simulink model "fu_simu_png_radome_directerror"  (R2020a)
settings: Solver=FixedStepAuto  StartTime=0.0  StopTime=20  FixedStep=0.001  RelTol=1e-3
values from neighbouring files (symbols this model uses):
  gamma_M_0 = deg2rad(0)    [initial.m]
  lambda_0 = deg2rad(5.7106)    [initial.m]
  N = 4    [initial.m]
  R_0 = 10050    [initial.m]
  T_alpha = 1    [initial.m]
  tau = 0.1    [initial.m]
  V_M = 500    [initial.m]
settings Model: Creator=anwaei  LastModifiedBy=anwaei

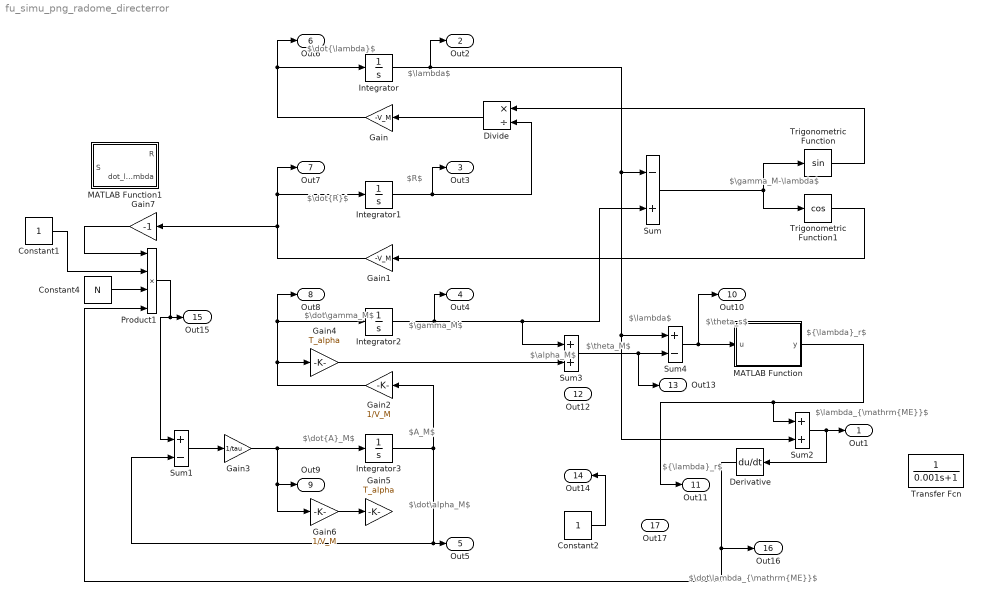
== system fu_simu_png_radome_directerror ==
  note: $\lambda$
  note: $R$
  note: $\gamma_M$
  note: $A_M$
  note: $\gamma_M-\lambda$
  note: $\dot{\lambda}$
  note: $\dot{R}$
  note: $\dot\gamma_M$
  note: $\dot{A}_M$
  note: $\alpha_M$
  note: $\theta_M$
  note: $\theta_s$
  note: $\dot\alpha_M$
  note: $\lambda$
  note: ${\lambda}_r$
  note: $\lambda_{\mathrm{ME}}$
  note: $\dot\lambda_{\mathrm{ME}}$
  note: ${\lambda}_r$
  Constant1 : Constant
  Constant2 : Constant
  Constant4 : Constant  Value=N
  Derivative : Derivative
  Divide : Product  Inputs=*/
  Gain : Gain  Gain=-V_M
  Gain1 : Gain  Gain=-V_M
  Gain2 : Gain  Gain=1/V_M
  Gain3 : Gain  Gain=1/tau
  Gain4 : Gain  Gain=T_alpha
  Gain5 : Gain  Gain=T_alpha
  Gain6 : Gain  Gain=1/V_M
  Gain7 : Gain  Gain=-1
  Integrator : Integrator  InitialCondition=lambda_0
  Integrator1 : Integrator  InitialCondition=R_0
  Integrator2 : Integrator  InitialCondition=gamma_M_0
  Integrator3 : Integrator
  MATLAB Function : MATLAB Function  TreatAsAtomicUnit=on
  MATLAB Function1 : MATLAB Function  TreatAsAtomicUnit=on
  Product1 : Product  Inputs=4
  Sum : Sum  Inputs=-+
  Sum1 : Sum  Inputs=+-
  Sum2 : Sum
  Sum3 : Sum
  Sum4 : Sum  Inputs=+-
  Transfer Fcn : TransferFcn  Denominator=[0.001 1]
  Trigonometric Function : Trigonometry
  Trigonometric Function1 : Trigonometry  Operator=cos
  Out1 : Outport
  Out2 : Outport  Port=2
  Out3 : Outport  Port=3
  Out4 : Outport  Port=4
  Out5 : Outport  Port=5
  Out6 : Outport  Port=6
  Out7 : Outport  Port=7
  Out8 : Outport  Port=8
  Out9 : Outport  Port=9
  Out10 : Outport  Port=10
  Out11 : Outport  Port=11
  Out12 : Outport  Port=12
  Out13 : Outport  Port=13
  Out14 : Outport  Port=14
  Out15 : Outport  Port=15
  Out16 : Outport  Port=16
  Out17 : Outport  Port=17
  wires:
  Integrator/1 -> Out2/1, Sum2/2, Sum4/1, Sum/1
  Integrator1/1 -> Out3/1, Divide/2
  Integrator2/1 -> Out4/1, Sum3/1, Sum/2
  Integrator3/1 -> Gain2/1, Sum1/2, Out5/1
  Sum/1 -> Trigonometric Function/1, Trigonometric Function1/1
  Trigonometric Function/1 -> Divide/1
  Divide/1 -> Gain/1
  Gain/1 -> Out6/1, Integrator/1
  Trigonometric Function1/1 -> Gain1/1
  Gain1/1 -> Gain7/1, Out7/1, Integrator1/1
  Gain2/1 -> Gain4/1, Out8/1, Integrator2/1
  Gain3/1 -> Out9/1, Gain6/1, Integrator3/1
  Sum3/1 -> Out13/1, Sum4/2
  Sum4/1 -> Out10/1, MATLAB Function/1(u)
  Gain6/1 -> Gain5/1
  MATLAB Function/1(y) -> Sum2/1, Out11/1
  Gain7/1 -> Product1/1
  Constant4/1 -> Product1/3
  Product1/1 -> Sum1/1, Out15/1
  Sum1/1 -> Gain3/1
  Sum2/1 -> Derivative/1, Out1/1
  Constant1/1 -> Product1/2
  Gain4/1 -> Sum3/2
  Derivative/1 -> Out16/1, Product1/4
  Constant2/1 -> Out14/1

== matlab function fu_simu_png_radome_directerror/MATLAB Function ==
  data: u input; y output
function y = fcn(u)

%%
r=deg2rad(-0.5);
zeta=4;
p=1;
y=r*exp(-zeta*abs(u))*sin(2*pi/p*u);

% if u<0
%     a=exp(zeta*u);
%     b=zeta*sin(2*pi*u/p);
%     c=2*pi/p*cos(2*pi*u/p);
% else
%     a=exp(-zeta*u);
%     b=-zeta*sin(2*pi*u/p);
%     c=2*pi/p*cos(2*pi*u/p);
% end
% 
% y=r*a*(b+c);
% y=y/rad2deg(1);

%%
% y=0.025;
% y=0.05;
% y=-0.025;

== matlab function fu_simu_png_radome_directerror/MATLAB Function1 ==
  settings: updateMethod=DISCRETE
  data: R input; S output; dot_lambda input
function S = fcn(R,dot_lambda)

k = 0.5;
R_0 = 10050;
persistent i miu_L miu_U S_previous

if isempty(i)
    i=1;
else
    i=i+1;
end

if isempty(miu_L)
    miu_L = deg2rad(0.5)/R_0^k;
end

if isempty(miu_U)
    miu_U = deg2rad(1.5)/R_0^k;
end

dot_lambda_L = miu_L * R^k;
dot_lambda_U = miu_L * R^k;

if isempty(S_previous)
    if abs(dot_lambda)>dot_lambda_L
        S = 0;
    else
        S = 1;
    end
    S_previous = S;
%     Ss = S;
else
    if abs(dot_lambda)>=dot_lambda_U
        S = 1;
    elseif abs(dot_lambda)>dot_lambda_L
%         S = Ss(i-1);
        S = S_previous;
    else
        S = 0;
    end
    S_previous = S;
%     Ss = [Ss S];
end

end
